simulink model "wip_main"  (R2024a)
settings: Solver=VariableStepAuto  StartTime=0.0  StopTime=1000  RelTol=1e-3
settings Model: Creator=filip  LastModifiedBy=filip

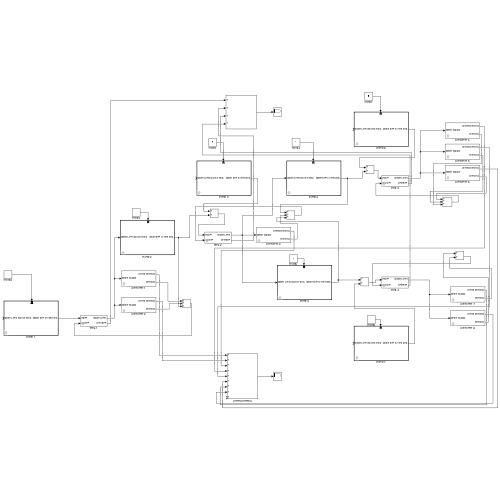
[thumbnail: Simulink's stored preview of the top-level diagram]
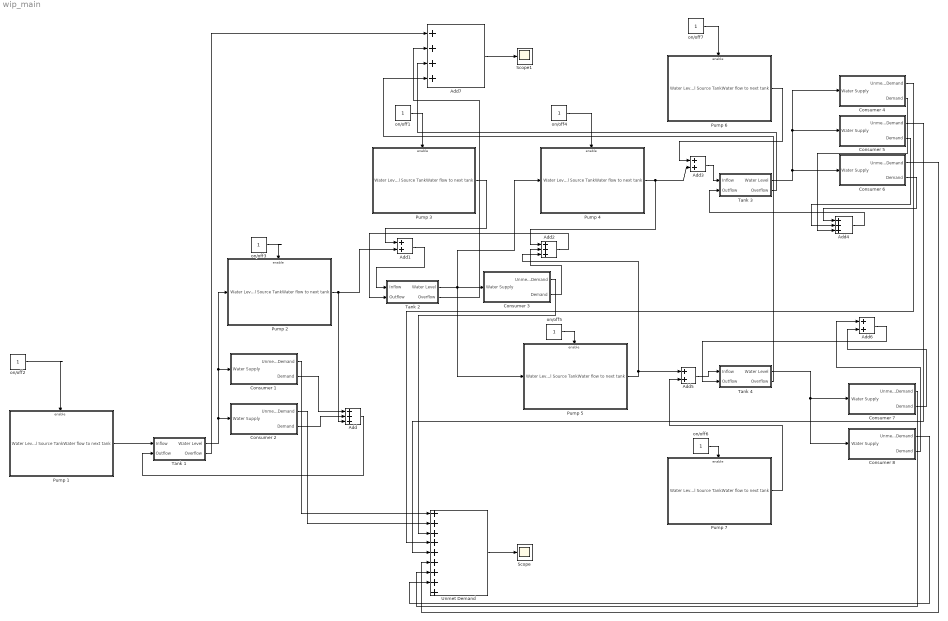
== system wip_main ==
  Add : Sum  Inputs=+++
  Add{1,3,5..6} (4 alike) : Sum
  Add2 : Sum  Inputs=+++
  Add4 : Sum  Inputs=+++
  Add7 : Sum  Inputs=++++
  Consumer 1 : Subsystem  mask{a_i=1, f_i=2, d_i=50}
      mask prompts: f_i "frequenz"; d_i "delay"
  Consumer 2 : Subsystem  mask{a_i=1, f_i=2, d_i=50}
      mask prompts: f_i "frequenz"; d_i "delay"
  Consumer 3 : Subsystem  mask{a_i=1, f_i=2, d_i=50}
      mask prompts: f_i "frequenz"; d_i "delay"
  Consumer 4 : Subsystem  mask{a_i=1, f_i=2, d_i=50}
      mask prompts: f_i "frequenz"; d_i "delay"
  Consumer 5 : Subsystem  mask{a_i=1, f_i=2, d_i=50}
      mask prompts: f_i "frequenz"; d_i "delay"
  Consumer 6 : Subsystem  mask{a_i=1, f_i=2, d_i=50}
      mask prompts: f_i "frequenz"; d_i "delay"
  Consumer 7 : Subsystem  mask{a_i=1, f_i=2, d_i=50}
      mask prompts: f_i "frequenz"; d_i "delay"
  Consumer 8 : Subsystem  mask{a_i=1, f_i=2, d_i=50}
      mask prompts: f_i "frequenz"; d_i "delay"
  Pump 1 : Subsystem  TreatAsAtomicUnit=on  mask{p_i=15}
      mask prompts: p_i "volume per Time (p_i)"
  Pump 2 : Subsystem  TreatAsAtomicUnit=on  mask{p_i=20}
      mask prompts: p_i "volume per Time (p_i)"
  Pump 3 : Subsystem  TreatAsAtomicUnit=on  mask{p_i=5}
      mask prompts: p_i "volume per Time (p_i)"
  Pump 4 : Subsystem  TreatAsAtomicUnit=on  mask{p_i=7}
      mask prompts: p_i "volume per Time (p_i)"
  Pump 5 : Subsystem  TreatAsAtomicUnit=on  mask{p_i=3}
      mask prompts: p_i "volume per Time (p_i)"
  Pump 6 : Subsystem  TreatAsAtomicUnit=on  mask{p_i=5}
      mask prompts: p_i "volume per Time (p_i)"
  Pump 7 : Subsystem  TreatAsAtomicUnit=on  mask{p_i=5}
      mask prompts: p_i "volume per Time (p_i)"
  Scope : Scope
  Scope1 : Scope
  Tank 1 : Subsystem  mask{c_i=100, c_i_init=50}
      mask prompts: c_i "capacity (c_i)"; c_i_init "Init capacity (c_i_init)"
  Tank 2 : Subsystem  mask{c_i=100, c_i_init=50}
      mask prompts: c_i "capacity (c_i)"; c_i_init "Init capacity (c_i_init)"
  Tank 3 : Subsystem  mask{c_i=100, c_i_init=50}
      mask prompts: c_i "capacity (c_i)"; c_i_init "Init capacity (c_i_init)"
  Tank 4 : Subsystem  mask{c_i=100, c_i_init=0}
      mask prompts: c_i "capacity (c_i)"; c_i_init "Init capacity (c_i_init)"
  Unmet Demand : Sum  Inputs=+++++++++
  on/off{1..7} (7 alike) : Constant
  wires:
  on/off2/1 -> Pump 1/Enable
  Pump 1/1(Water flow to next tank) -> Tank 1/1(Inflow)
  Consumer 1/2(Demand) -> Add/1
  Consumer 2/2(Demand) -> Add/2
  Add/1 -> Tank 1/2(Outflow)
  Tank 1/1(Water Level) -> Consumer 2/1(Water Supply), Pump 2/1(Water Level Source Tank), Consumer 1/1(Water Supply)
  on/off1/1 -> Pump 3/Enable
  on/off3/1 -> Pump 2/Enable
  Pump 2/1(Water flow to next tank) -> Add/3, Add1/2
  Pump 3/1(Water flow to next tank) -> Add1/1
  Add1/1 -> Tank 2/1(Inflow)
  Tank 2/1(Water Level) -> Consumer 3/1(Water Supply), Pump 5/1(Water Level Source Tank), Pump 4/1(Water Level Source Tank)
  Pump 4/1(Water flow to next tank) -> Add2/1, Add3/2
  Consumer 3/2(Demand) -> Add2/2
  Pump 5/1(Water flow to next tank) -> Add2/3, Add5/1
  Add2/1 -> Tank 2/2(Outflow)
  Pump 6/1(Water flow to next tank) -> Add3/1
  Add3/1 -> Tank 3/1(Inflow)
  Tank 3/1(Water Level) -> Consumer 6/1(Water Supply), Consumer 5/1(Water Supply), Consumer 4/1(Water Supply)
  Consumer 6/2(Demand) -> Add4/1
  Consumer 5/2(Demand) -> Add4/2
  Consumer 4/2(Demand) -> Add4/3
  Add4/1 -> Tank 3/2(Outflow)
  Pump 7/1(Water flow to next tank) -> Add5/2
  Add5/1 -> Tank 4/1(Inflow)
  Tank 4/1(Water Level) -> Consumer 8/1(Water Supply), Consumer 7/1(Water Supply)
  Consumer 7/2(Demand) -> Add6/2
  Consumer 8/2(Demand) -> Add6/1
  Add6/1 -> Tank 4/2(Outflow)
  on/off4/1 -> Pump 4/Enable
  on/off5/1 -> Pump 5/Enable
  on/off6/1 -> Pump 7/Enable
  on/off7/1 -> Pump 6/Enable
  Consumer 1/1(Unmet Demand) -> Unmet Demand/1
  Consumer 2/1(Unmet Demand) -> Unmet Demand/2
  Consumer 3/1(Unmet Demand) -> Unmet Demand/3
  Consumer 4/1(Unmet Demand) -> Unmet Demand/4
  Consumer 5/1(Unmet Demand) -> Unmet Demand/5
  Consumer 6/1(Unmet Demand) -> Unmet Demand/6
  Consumer 7/1(Unmet Demand) -> Unmet Demand/7
  Consumer 8/1(Unmet Demand) -> Unmet Demand/8
  Unmet Demand/1 -> Scope/1
  Tank 1/2(Overflow) -> Add7/1
  Tank 2/2(Overflow) -> Add7/2
  Tank 3/2(Overflow) -> Add7/3
  Tank 4/2(Overflow) -> Add7/4
  Add7/1 -> Scope1/1

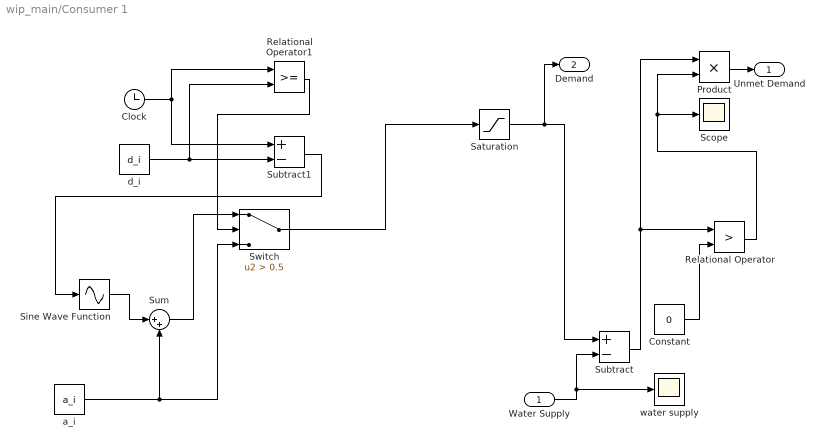
== system wip_main/Consumer 1 ==
  Water Supply : Inport
  Clock : Clock
  Constant : Constant  Value=0
  Product : Product
  Relational Operator : RelationalOperator  Operator=>  OutDataTypeStr=boolean  RndMeth=Simplest  InputSameDT=off
  Relational Operator1 : RelationalOperator  OutDataTypeStr=boolean  RndMeth=Simplest  InputSameDT=off
  Saturation : Saturate  UpperLimit=inf  LowerLimit=0
  Scope : Scope
  Sine Wave Function : Sin  TimeSource=Use external signal  Amplitude=a_i  Frequency=f_i  SampleTime=0
  Subtract : Sum  Inputs=+-
  Subtract1 : Sum  Inputs=+-
  Sum : Sum  Inputs=|++
  Switch : Switch  Criteria=u2 > Threshold  Threshold=0.5  SaturateOnIntegerOverflow=off  InputSameDT=off
  a_i : Constant  Value=a_i
  d_i : Constant  Value=d_i
  water supply : Scope
  Unmet Demand : Outport
  Demand : Outport  Port=2
  wires:
  a_i/1 -> Sum/2, Switch/3
  Water Supply/1 -> water supply/1, Subtract/2
  Subtract/1 -> Relational Operator/1, Product/1
  Relational Operator/1 -> Scope/1, Product/2
  Product/1 -> Unmet Demand/1
  Switch/1 -> Saturation/1
  Saturation/1 -> Demand/1, Subtract/1
  Constant/1 -> Relational Operator/2
  Clock/1 -> Relational Operator1/1, Subtract1/1
  d_i/1 -> Relational Operator1/2, Subtract1/2
  Subtract1/1 -> Sine Wave Function/1
  Relational Operator1/1 -> Switch/2
  Sum/1 -> Switch/1
  Sine Wave Function/1 -> Sum/1

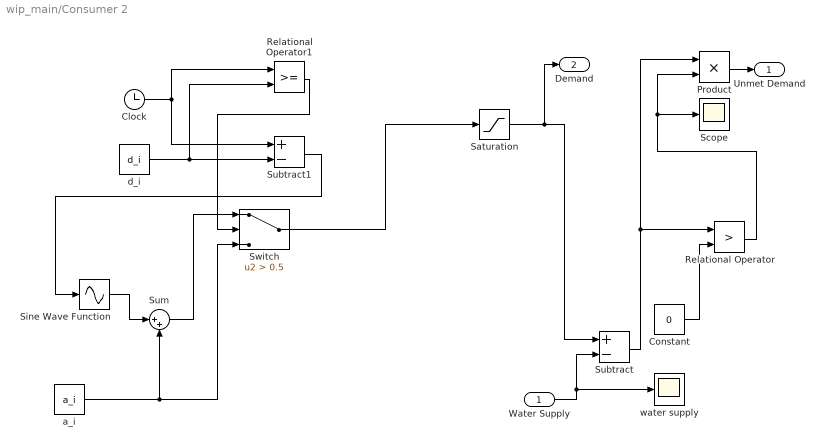
== system wip_main/Consumer 2 ==
  Water Supply : Inport
  Clock : Clock
  Constant : Constant  Value=0
  Product : Product
  Relational Operator : RelationalOperator  Operator=>  OutDataTypeStr=boolean  RndMeth=Simplest  InputSameDT=off
  Relational Operator1 : RelationalOperator  OutDataTypeStr=boolean  RndMeth=Simplest  InputSameDT=off
  Saturation : Saturate  UpperLimit=inf  LowerLimit=0
  Scope : Scope
  Sine Wave Function : Sin  TimeSource=Use external signal  Amplitude=a_i  Frequency=f_i  SampleTime=0
  Subtract : Sum  Inputs=+-
  Subtract1 : Sum  Inputs=+-
  Sum : Sum  Inputs=|++
  Switch : Switch  Criteria=u2 > Threshold  Threshold=0.5  SaturateOnIntegerOverflow=off  InputSameDT=off
  a_i : Constant  Value=a_i
  d_i : Constant  Value=d_i
  water supply : Scope
  Unmet Demand : Outport
  Demand : Outport  Port=2
  wires:
  a_i/1 -> Sum/2, Switch/3
  Water Supply/1 -> water supply/1, Subtract/2
  Subtract/1 -> Relational Operator/1, Product/1
  Relational Operator/1 -> Scope/1, Product/2
  Product/1 -> Unmet Demand/1
  Switch/1 -> Saturation/1
  Saturation/1 -> Demand/1, Subtract/1
  Constant/1 -> Relational Operator/2
  Clock/1 -> Relational Operator1/1, Subtract1/1
  d_i/1 -> Relational Operator1/2, Subtract1/2
  Subtract1/1 -> Sine Wave Function/1
  Relational Operator1/1 -> Switch/2
  Sum/1 -> Switch/1
  Sine Wave Function/1 -> Sum/1

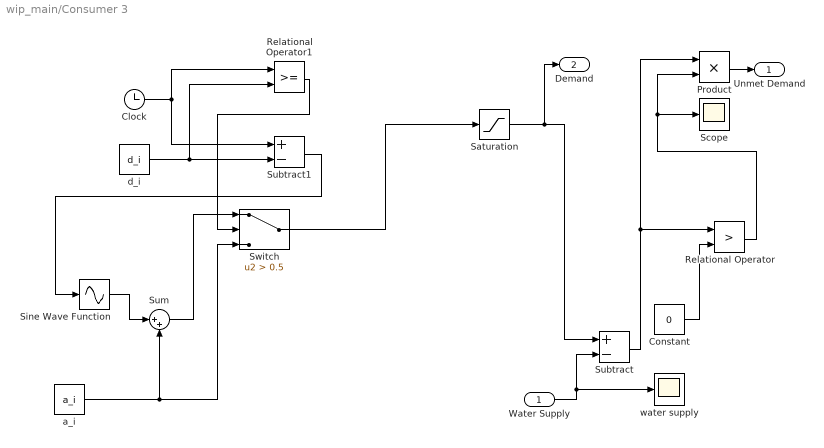
== system wip_main/Consumer 3 ==
  Water Supply : Inport
  Clock : Clock
  Constant : Constant  Value=0
  Product : Product
  Relational Operator : RelationalOperator  Operator=>  OutDataTypeStr=boolean  RndMeth=Simplest  InputSameDT=off
  Relational Operator1 : RelationalOperator  OutDataTypeStr=boolean  RndMeth=Simplest  InputSameDT=off
  Saturation : Saturate  UpperLimit=inf  LowerLimit=0
  Scope : Scope
  Sine Wave Function : Sin  TimeSource=Use external signal  Amplitude=a_i  Frequency=f_i  SampleTime=0
  Subtract : Sum  Inputs=+-
  Subtract1 : Sum  Inputs=+-
  Sum : Sum  Inputs=|++
  Switch : Switch  Criteria=u2 > Threshold  Threshold=0.5  SaturateOnIntegerOverflow=off  InputSameDT=off
  a_i : Constant  Value=a_i
  d_i : Constant  Value=d_i
  water supply : Scope
  Unmet Demand : Outport
  Demand : Outport  Port=2
  wires:
  a_i/1 -> Sum/2, Switch/3
  Water Supply/1 -> water supply/1, Subtract/2
  Subtract/1 -> Relational Operator/1, Product/1
  Relational Operator/1 -> Scope/1, Product/2
  Product/1 -> Unmet Demand/1
  Switch/1 -> Saturation/1
  Saturation/1 -> Demand/1, Subtract/1
  Constant/1 -> Relational Operator/2
  Clock/1 -> Relational Operator1/1, Subtract1/1
  d_i/1 -> Relational Operator1/2, Subtract1/2
  Subtract1/1 -> Sine Wave Function/1
  Relational Operator1/1 -> Switch/2
  Sum/1 -> Switch/1
  Sine Wave Function/1 -> Sum/1

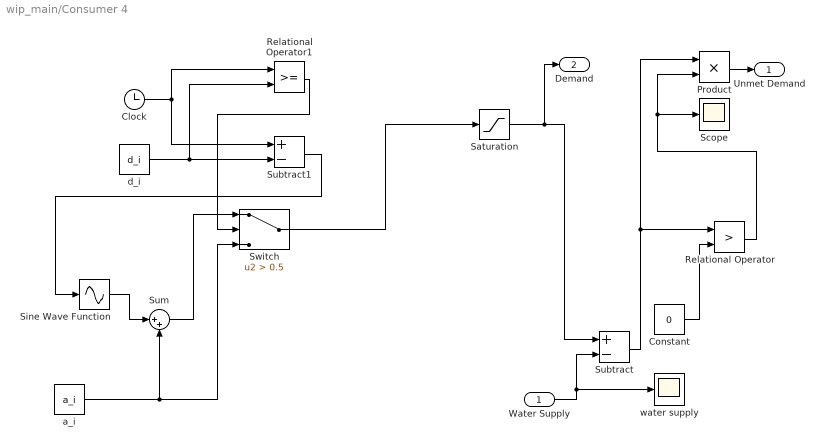
== system wip_main/Consumer 4 ==
  Water Supply : Inport
  Clock : Clock
  Constant : Constant  Value=0
  Product : Product
  Relational Operator : RelationalOperator  Operator=>  OutDataTypeStr=boolean  RndMeth=Simplest  InputSameDT=off
  Relational Operator1 : RelationalOperator  OutDataTypeStr=boolean  RndMeth=Simplest  InputSameDT=off
  Saturation : Saturate  UpperLimit=inf  LowerLimit=0
  Scope : Scope
  Sine Wave Function : Sin  TimeSource=Use external signal  Amplitude=a_i  Frequency=f_i  SampleTime=0
  Subtract : Sum  Inputs=+-
  Subtract1 : Sum  Inputs=+-
  Sum : Sum  Inputs=|++
  Switch : Switch  Criteria=u2 > Threshold  Threshold=0.5  SaturateOnIntegerOverflow=off  InputSameDT=off
  a_i : Constant  Value=a_i
  d_i : Constant  Value=d_i
  water supply : Scope
  Unmet Demand : Outport
  Demand : Outport  Port=2
  wires:
  a_i/1 -> Sum/2, Switch/3
  Water Supply/1 -> water supply/1, Subtract/2
  Subtract/1 -> Relational Operator/1, Product/1
  Relational Operator/1 -> Scope/1, Product/2
  Product/1 -> Unmet Demand/1
  Switch/1 -> Saturation/1
  Saturation/1 -> Demand/1, Subtract/1
  Constant/1 -> Relational Operator/2
  Clock/1 -> Relational Operator1/1, Subtract1/1
  d_i/1 -> Relational Operator1/2, Subtract1/2
  Subtract1/1 -> Sine Wave Function/1
  Relational Operator1/1 -> Switch/2
  Sum/1 -> Switch/1
  Sine Wave Function/1 -> Sum/1

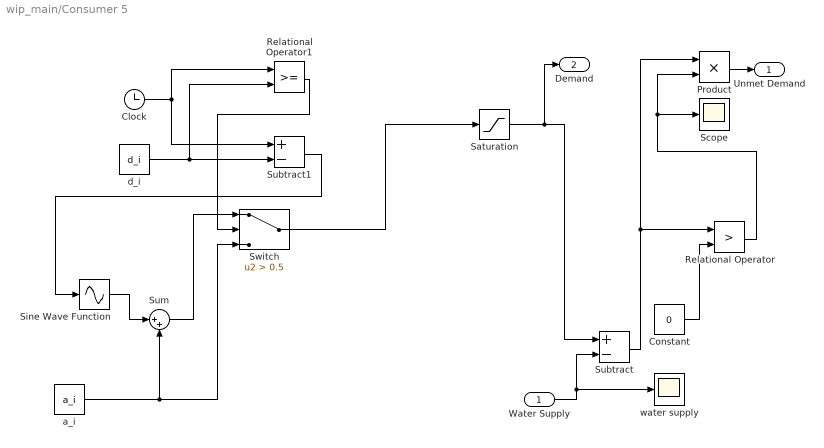
== system wip_main/Consumer 5 ==
  Water Supply : Inport
  Clock : Clock
  Constant : Constant  Value=0
  Product : Product
  Relational Operator : RelationalOperator  Operator=>  OutDataTypeStr=boolean  RndMeth=Simplest  InputSameDT=off
  Relational Operator1 : RelationalOperator  OutDataTypeStr=boolean  RndMeth=Simplest  InputSameDT=off
  Saturation : Saturate  UpperLimit=inf  LowerLimit=0
  Scope : Scope
  Sine Wave Function : Sin  TimeSource=Use external signal  Amplitude=a_i  Frequency=f_i  SampleTime=0
  Subtract : Sum  Inputs=+-
  Subtract1 : Sum  Inputs=+-
  Sum : Sum  Inputs=|++
  Switch : Switch  Criteria=u2 > Threshold  Threshold=0.5  SaturateOnIntegerOverflow=off  InputSameDT=off
  a_i : Constant  Value=a_i
  d_i : Constant  Value=d_i
  water supply : Scope
  Unmet Demand : Outport
  Demand : Outport  Port=2
  wires:
  a_i/1 -> Sum/2, Switch/3
  Water Supply/1 -> water supply/1, Subtract/2
  Subtract/1 -> Relational Operator/1, Product/1
  Relational Operator/1 -> Scope/1, Product/2
  Product/1 -> Unmet Demand/1
  Switch/1 -> Saturation/1
  Saturation/1 -> Demand/1, Subtract/1
  Constant/1 -> Relational Operator/2
  Clock/1 -> Relational Operator1/1, Subtract1/1
  d_i/1 -> Relational Operator1/2, Subtract1/2
  Subtract1/1 -> Sine Wave Function/1
  Relational Operator1/1 -> Switch/2
  Sum/1 -> Switch/1
  Sine Wave Function/1 -> Sum/1

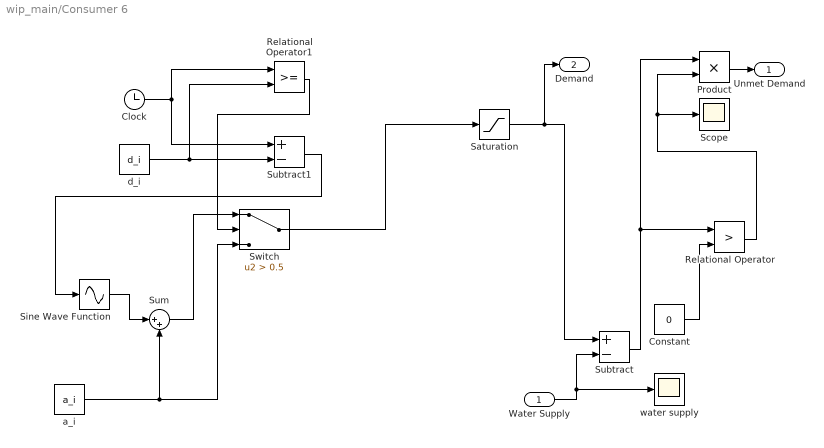
== system wip_main/Consumer 6 ==
  Water Supply : Inport
  Clock : Clock
  Constant : Constant  Value=0
  Product : Product
  Relational Operator : RelationalOperator  Operator=>  OutDataTypeStr=boolean  RndMeth=Simplest  InputSameDT=off
  Relational Operator1 : RelationalOperator  OutDataTypeStr=boolean  RndMeth=Simplest  InputSameDT=off
  Saturation : Saturate  UpperLimit=inf  LowerLimit=0
  Scope : Scope
  Sine Wave Function : Sin  TimeSource=Use external signal  Amplitude=a_i  Frequency=f_i  SampleTime=0
  Subtract : Sum  Inputs=+-
  Subtract1 : Sum  Inputs=+-
  Sum : Sum  Inputs=|++
  Switch : Switch  Criteria=u2 > Threshold  Threshold=0.5  SaturateOnIntegerOverflow=off  InputSameDT=off
  a_i : Constant  Value=a_i
  d_i : Constant  Value=d_i
  water supply : Scope
  Unmet Demand : Outport
  Demand : Outport  Port=2
  wires:
  a_i/1 -> Sum/2, Switch/3
  Water Supply/1 -> water supply/1, Subtract/2
  Subtract/1 -> Relational Operator/1, Product/1
  Relational Operator/1 -> Scope/1, Product/2
  Product/1 -> Unmet Demand/1
  Switch/1 -> Saturation/1
  Saturation/1 -> Demand/1, Subtract/1
  Constant/1 -> Relational Operator/2
  Clock/1 -> Relational Operator1/1, Subtract1/1
  d_i/1 -> Relational Operator1/2, Subtract1/2
  Subtract1/1 -> Sine Wave Function/1
  Relational Operator1/1 -> Switch/2
  Sum/1 -> Switch/1
  Sine Wave Function/1 -> Sum/1

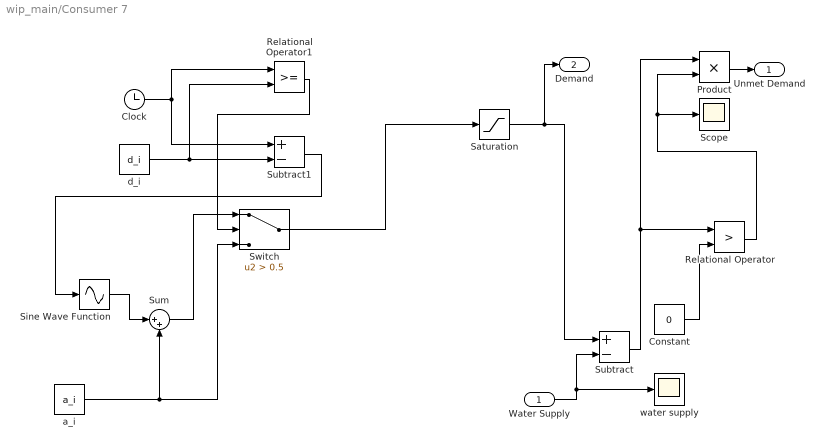
== system wip_main/Consumer 7 ==
  Water Supply : Inport
  Clock : Clock
  Constant : Constant  Value=0
  Product : Product
  Relational Operator : RelationalOperator  Operator=>  OutDataTypeStr=boolean  RndMeth=Simplest  InputSameDT=off
  Relational Operator1 : RelationalOperator  OutDataTypeStr=boolean  RndMeth=Simplest  InputSameDT=off
  Saturation : Saturate  UpperLimit=inf  LowerLimit=0
  Scope : Scope
  Sine Wave Function : Sin  TimeSource=Use external signal  Amplitude=a_i  Frequency=f_i  SampleTime=0
  Subtract : Sum  Inputs=+-
  Subtract1 : Sum  Inputs=+-
  Sum : Sum  Inputs=|++
  Switch : Switch  Criteria=u2 > Threshold  Threshold=0.5  SaturateOnIntegerOverflow=off  InputSameDT=off
  a_i : Constant  Value=a_i
  d_i : Constant  Value=d_i
  water supply : Scope
  Unmet Demand : Outport
  Demand : Outport  Port=2
  wires:
  a_i/1 -> Sum/2, Switch/3
  Water Supply/1 -> water supply/1, Subtract/2
  Subtract/1 -> Relational Operator/1, Product/1
  Relational Operator/1 -> Scope/1, Product/2
  Product/1 -> Unmet Demand/1
  Switch/1 -> Saturation/1
  Saturation/1 -> Demand/1, Subtract/1
  Constant/1 -> Relational Operator/2
  Clock/1 -> Relational Operator1/1, Subtract1/1
  d_i/1 -> Relational Operator1/2, Subtract1/2
  Subtract1/1 -> Sine Wave Function/1
  Relational Operator1/1 -> Switch/2
  Sum/1 -> Switch/1
  Sine Wave Function/1 -> Sum/1

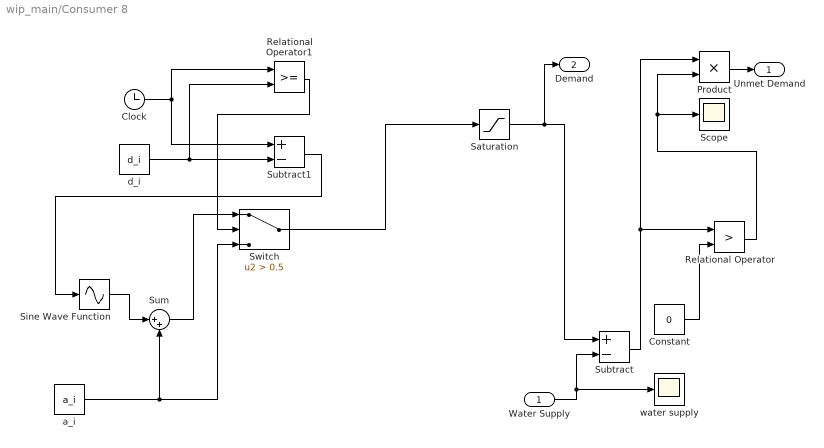
== system wip_main/Consumer 8 ==
  Water Supply : Inport
  Clock : Clock
  Constant : Constant  Value=0
  Product : Product
  Relational Operator : RelationalOperator  Operator=>  OutDataTypeStr=boolean  RndMeth=Simplest  InputSameDT=off
  Relational Operator1 : RelationalOperator  OutDataTypeStr=boolean  RndMeth=Simplest  InputSameDT=off
  Saturation : Saturate  UpperLimit=inf  LowerLimit=0
  Scope : Scope
  Sine Wave Function : Sin  TimeSource=Use external signal  Amplitude=a_i  Frequency=f_i  SampleTime=0
  Subtract : Sum  Inputs=+-
  Subtract1 : Sum  Inputs=+-
  Sum : Sum  Inputs=|++
  Switch : Switch  Criteria=u2 > Threshold  Threshold=0.5  SaturateOnIntegerOverflow=off  InputSameDT=off
  a_i : Constant  Value=a_i
  d_i : Constant  Value=d_i
  water supply : Scope
  Unmet Demand : Outport
  Demand : Outport  Port=2
  wires:
  a_i/1 -> Sum/2, Switch/3
  Water Supply/1 -> water supply/1, Subtract/2
  Subtract/1 -> Relational Operator/1, Product/1
  Relational Operator/1 -> Scope/1, Product/2
  Product/1 -> Unmet Demand/1
  Switch/1 -> Saturation/1
  Saturation/1 -> Demand/1, Subtract/1
  Constant/1 -> Relational Operator/2
  Clock/1 -> Relational Operator1/1, Subtract1/1
  d_i/1 -> Relational Operator1/2, Subtract1/2
  Subtract1/1 -> Sine Wave Function/1
  Relational Operator1/1 -> Switch/2
  Sum/1 -> Switch/1
  Sine Wave Function/1 -> Sum/1

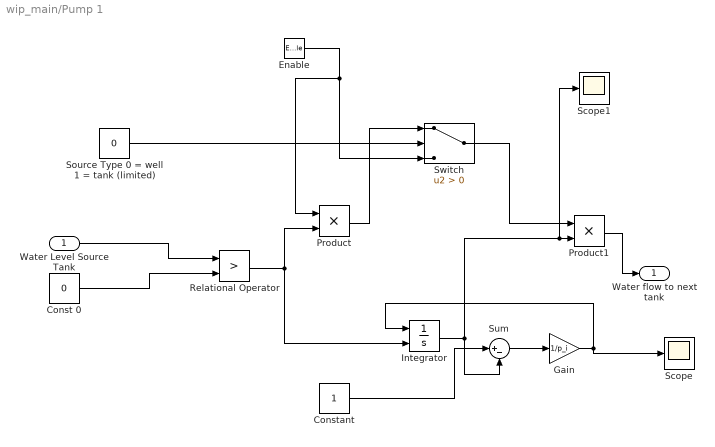
== system wip_main/Pump 1 ==
  Water Level Source Tank : Inport
  Enable : EnablePort  ShowOutputPort=on
  Const 0 : Constant  Value=0
  Constant : Constant
  Gain : Gain  Gain=1/p_i
  Integrator : Integrator  ExternalReset=falling
  Product : Product
  Product1 : Product
  Relational Operator : RelationalOperator  Operator=>  OutDataTypeStr=boolean  RndMeth=Simplest  InputSameDT=off
  Scope : Scope
  Scope1 : Scope
  Source Type 0 = well 1 = tank (limited) : Constant  Value=0
  Sum : Sum  Inputs=|+-
  Switch : Switch  Criteria=u2 > Threshold  SaturateOnIntegerOverflow=off  InputSameDT=off
  Water flow to next tank : Outport
  wires:
  Sum/1 -> Gain/1
  Integrator/1 -> Sum/2, Scope1/1, Product1/2
  Constant/1 -> Sum/1
  Gain/1 -> Scope/1, Integrator/1
  Enable/1 -> Switch/3, Product/1
  Source Type 0 = well 1 = tank (limited)/1 -> Switch/2
  Water Level Source Tank/1 -> Relational Operator/1
  Const 0/1 -> Relational Operator/2
  Relational Operator/1 -> Integrator/2, Product/2
  Product1/1 -> Water flow to next tank/1
  Switch/1 -> Product1/1
  Product/1 -> Switch/1

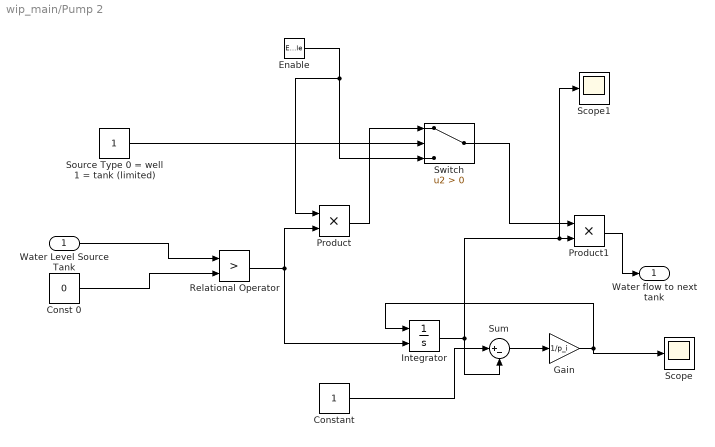
== system wip_main/Pump 2 ==
  Water Level Source Tank : Inport
  Enable : EnablePort  ShowOutputPort=on
  Const 0 : Constant  Value=0
  Constant : Constant
  Gain : Gain  Gain=1/p_i
  Integrator : Integrator  ExternalReset=falling
  Product : Product
  Product1 : Product
  Relational Operator : RelationalOperator  Operator=>  OutDataTypeStr=boolean  RndMeth=Simplest  InputSameDT=off
  Scope : Scope
  Scope1 : Scope
  Source Type 0 = well 1 = tank (limited) : Constant
  Sum : Sum  Inputs=|+-
  Switch : Switch  Criteria=u2 > Threshold  SaturateOnIntegerOverflow=off  InputSameDT=off
  Water flow to next tank : Outport
  wires:
  Sum/1 -> Gain/1
  Integrator/1 -> Sum/2, Scope1/1, Product1/2
  Constant/1 -> Sum/1
  Gain/1 -> Scope/1, Integrator/1
  Enable/1 -> Switch/3, Product/1
  Source Type 0 = well 1 = tank (limited)/1 -> Switch/2
  Water Level Source Tank/1 -> Relational Operator/1
  Const 0/1 -> Relational Operator/2
  Relational Operator/1 -> Integrator/2, Product/2
  Product1/1 -> Water flow to next tank/1
  Switch/1 -> Product1/1
  Product/1 -> Switch/1

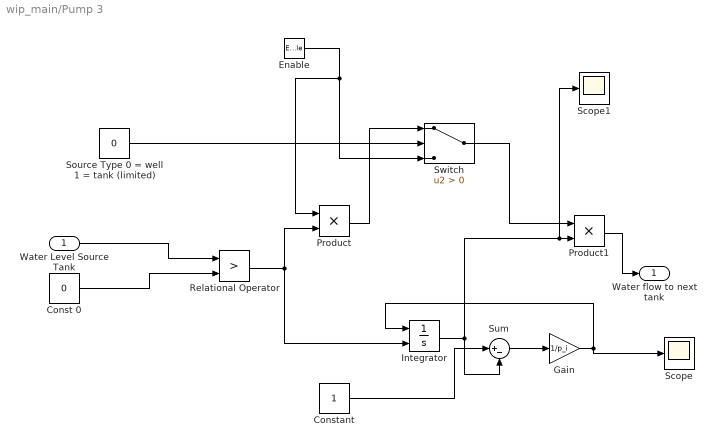
== system wip_main/Pump 3 ==
  Water Level Source Tank : Inport
  Enable : EnablePort  ShowOutputPort=on
  Const 0 : Constant  Value=0
  Constant : Constant
  Gain : Gain  Gain=1/p_i
  Integrator : Integrator  ExternalReset=falling
  Product : Product
  Product1 : Product
  Relational Operator : RelationalOperator  Operator=>  OutDataTypeStr=boolean  RndMeth=Simplest  InputSameDT=off
  Scope : Scope
  Scope1 : Scope
  Source Type 0 = well 1 = tank (limited) : Constant  Value=0
  Sum : Sum  Inputs=|+-
  Switch : Switch  Criteria=u2 > Threshold  SaturateOnIntegerOverflow=off  InputSameDT=off
  Water flow to next tank : Outport
  wires:
  Sum/1 -> Gain/1
  Integrator/1 -> Sum/2, Scope1/1, Product1/2
  Constant/1 -> Sum/1
  Gain/1 -> Scope/1, Integrator/1
  Enable/1 -> Switch/3, Product/1
  Source Type 0 = well 1 = tank (limited)/1 -> Switch/2
  Water Level Source Tank/1 -> Relational Operator/1
  Const 0/1 -> Relational Operator/2
  Relational Operator/1 -> Integrator/2, Product/2
  Product1/1 -> Water flow to next tank/1
  Switch/1 -> Product1/1
  Product/1 -> Switch/1

== system wip_main/Pump 4 ==
  Water Level Source Tank : Inport
  Enable : EnablePort  ShowOutputPort=on
  Const 0 : Constant  Value=0
  Constant : Constant
  Gain : Gain  Gain=1/p_i
  Integrator : Integrator  ExternalReset=falling
  Product : Product
  Product1 : Product
  Relational Operator : RelationalOperator  Operator=>  OutDataTypeStr=boolean  RndMeth=Simplest  InputSameDT=off
  Scope : Scope
  Scope1 : Scope
  Source Type 0 = well 1 = tank (limited) : Constant  Value=0
  Sum : Sum  Inputs=|+-
  Switch : Switch  Criteria=u2 > Threshold  SaturateOnIntegerOverflow=off  InputSameDT=off
  Water flow to next tank : Outport
  wires:
  Sum/1 -> Gain/1
  Integrator/1 -> Sum/2, Scope1/1, Product1/2
  Constant/1 -> Sum/1
  Gain/1 -> Scope/1, Integrator/1
  Enable/1 -> Switch/3, Product/1
  Source Type 0 = well 1 = tank (limited)/1 -> Switch/2
  Water Level Source Tank/1 -> Relational Operator/1
  Const 0/1 -> Relational Operator/2
  Relational Operator/1 -> Integrator/2, Product/2
  Product1/1 -> Water flow to next tank/1
  Switch/1 -> Product1/1
  Product/1 -> Switch/1

== system wip_main/Pump 5 ==
  Water Level Source Tank : Inport
  Enable : EnablePort  ShowOutputPort=on
  Const 0 : Constant  Value=0
  Constant : Constant
  Gain : Gain  Gain=1/p_i
  Integrator : Integrator  ExternalReset=falling
  Product : Product
  Product1 : Product
  Relational Operator : RelationalOperator  Operator=>  OutDataTypeStr=boolean  RndMeth=Simplest  InputSameDT=off
  Scope : Scope
  Scope1 : Scope
  Source Type 0 = well 1 = tank (limited) : Constant  Value=0
  Sum : Sum  Inputs=|+-
  Switch : Switch  Criteria=u2 > Threshold  SaturateOnIntegerOverflow=off  InputSameDT=off
  Water flow to next tank : Outport
  wires:
  Sum/1 -> Gain/1
  Integrator/1 -> Sum/2, Scope1/1, Product1/2
  Constant/1 -> Sum/1
  Gain/1 -> Scope/1, Integrator/1
  Enable/1 -> Switch/3, Product/1
  Source Type 0 = well 1 = tank (limited)/1 -> Switch/2
  Water Level Source Tank/1 -> Relational Operator/1
  Const 0/1 -> Relational Operator/2
  Relational Operator/1 -> Integrator/2, Product/2
  Product1/1 -> Water flow to next tank/1
  Switch/1 -> Product1/1
  Product/1 -> Switch/1

== system wip_main/Pump 6 ==
  Water Level Source Tank : Inport
  Enable : EnablePort  ShowOutputPort=on
  Const 0 : Constant  Value=0
  Constant : Constant
  Gain : Gain  Gain=1/p_i
  Integrator : Integrator  ExternalReset=falling
  Product : Product
  Product1 : Product
  Relational Operator : RelationalOperator  Operator=>  OutDataTypeStr=boolean  RndMeth=Simplest  InputSameDT=off
  Scope : Scope
  Scope1 : Scope
  Source Type 0 = well 1 = tank (limited) : Constant  Value=0
  Sum : Sum  Inputs=|+-
  Switch : Switch  Criteria=u2 > Threshold  SaturateOnIntegerOverflow=off  InputSameDT=off
  Water flow to next tank : Outport
  wires:
  Sum/1 -> Gain/1
  Integrator/1 -> Sum/2, Scope1/1, Product1/2
  Constant/1 -> Sum/1
  Gain/1 -> Scope/1, Integrator/1
  Enable/1 -> Switch/3, Product/1
  Source Type 0 = well 1 = tank (limited)/1 -> Switch/2
  Water Level Source Tank/1 -> Relational Operator/1
  Const 0/1 -> Relational Operator/2
  Relational Operator/1 -> Integrator/2, Product/2
  Product1/1 -> Water flow to next tank/1
  Switch/1 -> Product1/1
  Product/1 -> Switch/1

== system wip_main/Pump 7 ==
  Water Level Source Tank : Inport
  Enable : EnablePort  ShowOutputPort=on
  Const 0 : Constant  Value=0
  Constant : Constant
  Gain : Gain  Gain=1/p_i
  Integrator : Integrator  ExternalReset=falling
  Product : Product
  Product1 : Product
  Relational Operator : RelationalOperator  Operator=>  OutDataTypeStr=boolean  RndMeth=Simplest  InputSameDT=off
  Scope : Scope
  Scope1 : Scope
  Source Type 0 = well 1 = tank (limited) : Constant  Value=0
  Sum : Sum  Inputs=|+-
  Switch : Switch  Criteria=u2 > Threshold  SaturateOnIntegerOverflow=off  InputSameDT=off
  Water flow to next tank : Outport
  wires:
  Sum/1 -> Gain/1
  Integrator/1 -> Sum/2, Scope1/1, Product1/2
  Constant/1 -> Sum/1
  Gain/1 -> Scope/1, Integrator/1
  Enable/1 -> Switch/3, Product/1
  Source Type 0 = well 1 = tank (limited)/1 -> Switch/2
  Water Level Source Tank/1 -> Relational Operator/1
  Const 0/1 -> Relational Operator/2
  Relational Operator/1 -> Integrator/2, Product/2
  Product1/1 -> Water flow to next tank/1
  Switch/1 -> Product1/1
  Product/1 -> Switch/1

== system wip_main/Tank 1 ==
  Inflow : Inport
  Outflow : Inport  Port=2
  Capacity c_i : Constant  Value=c_i
  Gain : Gain
  "Initial Waterlevel c_i, init" : Constant  Value=c_i_init
  Integrator : Integrator  InitialConditionSource=external
  Product : Product
  Relational Operator : RelationalOperator  Operator=>  OutDataTypeStr=boolean  RndMeth=Simplest  InputSameDT=off
  Saturation : Saturate  UpperLimit=100  LowerLimit=0
  Subtract : Sum  Inputs=+-
  Sum : Sum  Inputs=|+-
  Water Level : Outport
  Overflow : Outport  Port=2
  wires:
  Inflow/1 -> Sum/1
  Outflow/1 -> Sum/2
  Sum/1 -> Integrator/1
  Integrator/1 -> Gain/1
  Gain/1 -> Relational Operator/1, Subtract/1, Saturation/1
  Capacity c_i/1 -> Relational Operator/2, Subtract/2
  Saturation/1 -> Water Level/1
  Product/1 -> Overflow/1
  Subtract/1 -> Product/1
  Relational Operator/1 -> Product/2
  "Initial Waterlevel c_i, init"/1 -> Integrator/2

== system wip_main/Tank 2 ==
  Inflow : Inport
  Outflow : Inport  Port=2
  Capacity c_i : Constant  Value=c_i
  Gain : Gain
  "Initial Waterlevel c_i, init" : Constant  Value=c_i_init
  Integrator : Integrator  InitialConditionSource=external
  Product : Product
  Relational Operator : RelationalOperator  Operator=>  OutDataTypeStr=boolean  RndMeth=Simplest  InputSameDT=off
  Saturation : Saturate  UpperLimit=100  LowerLimit=0
  Subtract : Sum  Inputs=+-
  Sum : Sum  Inputs=|+-
  Water Level : Outport
  Overflow : Outport  Port=2
  wires:
  Inflow/1 -> Sum/1
  Outflow/1 -> Sum/2
  Sum/1 -> Integrator/1
  Integrator/1 -> Gain/1
  Gain/1 -> Relational Operator/1, Subtract/1, Saturation/1
  Capacity c_i/1 -> Relational Operator/2, Subtract/2
  Saturation/1 -> Water Level/1
  Product/1 -> Overflow/1
  Subtract/1 -> Product/1
  Relational Operator/1 -> Product/2
  "Initial Waterlevel c_i, init"/1 -> Integrator/2

== system wip_main/Tank 3 ==
  Inflow : Inport
  Outflow : Inport  Port=2
  Capacity c_i : Constant  Value=c_i
  Gain : Gain
  "Initial Waterlevel c_i, init" : Constant  Value=c_i_init
  Integrator : Integrator  InitialConditionSource=external
  Product : Product
  Relational Operator : RelationalOperator  Operator=>  OutDataTypeStr=boolean  RndMeth=Simplest  InputSameDT=off
  Saturation : Saturate  UpperLimit=100  LowerLimit=0
  Subtract : Sum  Inputs=+-
  Sum : Sum  Inputs=|+-
  Water Level : Outport
  Overflow : Outport  Port=2
  wires:
  Inflow/1 -> Sum/1
  Outflow/1 -> Sum/2
  Sum/1 -> Integrator/1
  Integrator/1 -> Gain/1
  Gain/1 -> Relational Operator/1, Subtract/1, Saturation/1
  Capacity c_i/1 -> Relational Operator/2, Subtract/2
  Saturation/1 -> Water Level/1
  Product/1 -> Overflow/1
  Subtract/1 -> Product/1
  Relational Operator/1 -> Product/2
  "Initial Waterlevel c_i, init"/1 -> Integrator/2

== system wip_main/Tank 4 ==
  Inflow : Inport
  Outflow : Inport  Port=2
  Capacity c_i : Constant  Value=c_i
  Gain : Gain
  "Initial Waterlevel c_i, init" : Constant  Value=c_i_init
  Integrator : Integrator  InitialConditionSource=external
  Product : Product
  Relational Operator : RelationalOperator  Operator=>  OutDataTypeStr=boolean  RndMeth=Simplest  InputSameDT=off
  Saturation : Saturate  UpperLimit=100  LowerLimit=0
  Subtract : Sum  Inputs=+-
  Sum : Sum  Inputs=|+-
  Water Level : Outport
  Overflow : Outport  Port=2
  wires:
  Inflow/1 -> Sum/1
  Outflow/1 -> Sum/2
  Sum/1 -> Integrator/1
  Integrator/1 -> Gain/1
  Gain/1 -> Relational Operator/1, Subtract/1, Saturation/1
  Capacity c_i/1 -> Relational Operator/2, Subtract/2
  Saturation/1 -> Water Level/1
  Product/1 -> Overflow/1
  Subtract/1 -> Product/1
  Relational Operator/1 -> Product/2
  "Initial Waterlevel c_i, init"/1 -> Integrator/2
